simulink model "FOBReceiver"  (R2023b)
settings: Solver=VariableStepAuto  StartTime=0.0  StopTime=10.0  RelTol=1e-3
settings Model: DataDictionary=Interfaces.sldd  Creator=The MathWorks, Inc.  LastModifiedBy=The MathWorks, Inc.
settings SolverCC: AlgebraicLoopSolver=TrustRegion
settings DebuggingCC: UnconnectedInputMsg=warning  UnconnectedOutputMsg=warning  UnconnectedLineMsg=warning  SymbolicDimsDataTypeCodeGenerationDiagnostic=none
settings ModelReferenceCC: EnableRefExpFcnMdlSchedulingChecks=on

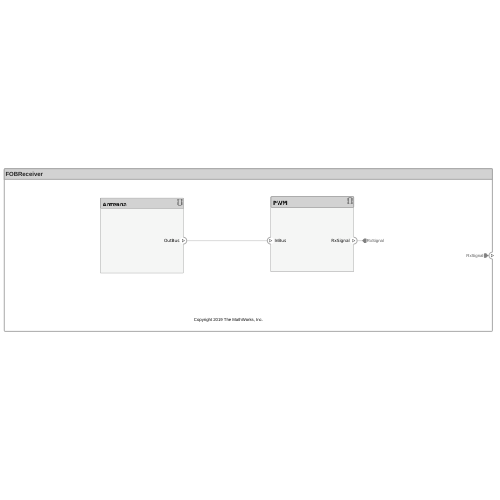
[thumbnail: Simulink's stored preview of the top-level diagram]
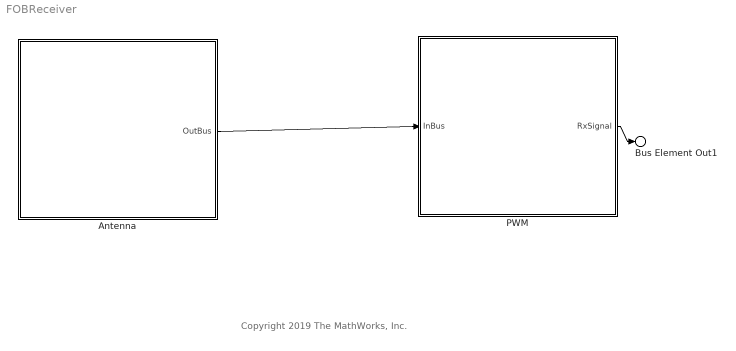
== system FOBReceiver ==
  note: Copyright 2019 The MathWorks, Inc.
  Antenna : Subsystem
      settings: PortSchema="{\"entries\":[{\"content\":{\"headerSize\":26,\"margin\":15,\"minimumSpacing\":25,\"sides\":[{\"content\":{\"connectorIds\":[]},\"type\":\"ConnectorPlacement.EquallySpacedRectSide\",\"uuid\":\"a0f82e88-5275-4bb9-87fe-a49bf19782cf\"},{\"content\":{\"connectorIds\":[\"Out1\"],\"side\":\"RIGHT\"},\"type\":\"ConnectorPlacement.EquallySpacedRectSide\",\"uuid\":\"4b3945c4-3891-41a7-b741-bb467a4ccb5a\"},{\"content\":{\"connectorIds\":[],\"side\":\"TOP\"},\"type\":\"ConnectorPlacement.EquallySpacedRectSide\",\"uuid\":\"042b1b4e-e1cf-4b0e-a9d9-106bb99a7cf5\"}]},\"type\":\"ConnectorPlacement.EquallySpacedConnector\",\"uuid\":\"79d888da-39cf-4e1d-aa7b-1e8818e96d62\"}],\"packageUris\":[\"http://schema.mathworks.com/mf0/Connector/19700101\"],\"version\":\"1.0\"}"
  PWM : Subsystem
      settings: PortSchema="{\"entries\":[{\"content\":{\"headerSize\":26,\"margin\":15,\"minimumSpacing\":25,\"sides\":[{\"content\":{\"connectorIds\":[\"In1\"]},\"type\":\"ConnectorPlacement.EquallySpacedRectSide\",\"uuid\":\"a0f82e88-5275-4bb9-87fe-a49bf19782cf\"},{\"content\":{\"connectorIds\":[\"Out1\"],\"side\":\"RIGHT\"},\"type\":\"ConnectorPlacement.EquallySpacedRectSide\",\"uuid\":\"4b3945c4-3891-41a7-b741-bb467a4ccb5a\"},{\"content\":{\"connectorIds\":[],\"side\":\"TOP\"},\"type\":\"ConnectorPlacement.EquallySpacedRectSide\",\"uuid\":\"042b1b4e-e1cf-4b0e-a9d9-106bb99a7cf5\"}]},\"type\":\"ConnectorPlacement.EquallySpacedConnector\",\"uuid\":\"79d888da-39cf-4e1d-aa7b-1e8818e96d62\"}],\"packageUris\":[\"http://schema.mathworks.com/mf0/Connector/19700101\"],\"version\":\"1.0\"}"
  Bus Element Out1 : Outport  PortName=RxSignal
  wires:
  Antenna/1(OutBus) -> PWM/1(InBus)
  PWM/1(RxSignal) -> Bus Element Out1/1

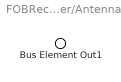
== system FOBReceiver/Antenna ==
  Bus Element Out1 : Outport  PortName=OutBus

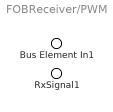
== system FOBReceiver/PWM ==
  Bus Element In1 : Inport  PortName=InBus
  RxSignal1 : Outport  PortName=RxSignal
